simulink model "MPC_Experiments_2"  (R2020a)
settings: Solver=FixedStepAuto  StartTime=0.0  StopTime=tsim  FixedStep=baseRate  RelTol=1e-3  EnableMultiTasking=on
values from neighbouring files (symbols this model uses):
  Ad = dss.A    [theInitializer.m]
  ALGORITHM = 5    [Run_Initializer.m]    (also in main.m)
  baseRate = 0.05    [Run_Initializer.m]
  Bd = dss.B    [theInitializer.m]
  Cmat = zeros(6*N,9*N)    [theInitializer.m]
  con0 = [n*N, 2*N, N, N, N, N]    [Run_Initializer.m]    (also in main.m)
  drop_states_BLACK = rand([3,1])/10+init_states_BLACK    [Run_Initializer.m]
  drop_states_BLUE = rand([3,1])/10+init_states_BLUE    [Run_Initializer.m]
  drop_states_RED = rand([3,1])/10+init_states_RED    [Run_Initializer.m]
  F_thrusters_BLACK = 0.25.*ones(8,1)    [Run_Initializer.m]
  F_thrusters_BLUE = 0.25.*ones(8,1)    [Run_Initializer.m]
  F_thrusters_RED = 0.25.*ones(8,1)    [Run_Initializer.m]
  Fmat = reshape(repmat([umax,umax,taumax],N,1),3*N,1)    [theInitializer.m]
  gamma = 0.95    [theInitializer.m]
  H = blkdiag(pattern{:})    [theInitializer.m]
  home_states_BLACK = [ xLength/2; yLength/2; 0]    [Run_Initializer.m]
  home_states_BLUE = [ xLength/2-0.9; yLength/2+0.5; 0]    [Run_Initializer.m]
  home_states_RED = [ xLength/2+0.7; yLength/2; pi]    [Run_Initializer.m]
  init_states_BLACK = [ct;thetat0]    [Run_Initializer.m]
  init_states_BLUE = [pobj1;0]    [Run_Initializer.m]
  init_states_RED = xi(1:3)    [Run_Initializer.m]
  Kd_tb = 0.4    [Run_Initializer.m]
  Kd_tblue = 0.4    [Run_Initializer.m]
  Kd_tr = 0.4    [Run_Initializer.m]
  Kd_xb = 5    [Run_Initializer.m]
  Kd_xblue = 5    [Run_Initializer.m]
  Kd_xr = 5    [Run_Initializer.m]
  Kd_yb = 5    [Run_Initializer.m]
  Kd_yblue = 5    [Run_Initializer.m]
  Kd_yr = 5    [Run_Initializer.m]
  KOZ_actual = KOZ + rc*sqrt(2)    [theInitializer.m]
  Kp_tb = 0.1    [Run_Initializer.m]
  Kp_tblue = 0.1    [Run_Initializer.m]
  Kp_tr = 0.1    [Run_Initializer.m]
  Kp_xb = 2    [Run_Initializer.m]
  Kp_xblue = 2    [Run_Initializer.m]
  Kp_xr = 2    [Run_Initializer.m]
  Kp_yb = 2    [Run_Initializer.m]
  Kp_yblue = 2    [Run_Initializer.m]
  Kp_yr = 2    [Run_Initializer.m]
  N = 15    [Run_Initializer.m]    (also in main.m)
  noise_variance_BLACK = 0    [Run_Initializer.m]
  noise_variance_BLUE = 0    [Run_Initializer.m]
  noise_variance_RED = 0    [Run_Initializer.m]
  Phase0_End = Phase0_Duration    (= 5)    [Run_Initializer.m]
  Phase1_End = Phase0_Duration + Phase1_Duration    (= 10)    [Run_Initializer.m]
  Phase2_End = Phase0_Duration + Phase1_Duration +                                   Phase2_Duration    (= 36)    [Run_Initializer.m]
  Phase3_End = Phase0_Duration + Phase1_Duration +                                   Phase2_Duration + Phase3_Duration    (= 166)    [Run_Initializer.m]
  Phase3_SubPhase1_End = Phase2_End + Phase3_SubPhase1_Duration    (= 40)    [Run_Initializer.m]
  Phase3_SubPhase2_End = Phase2_End + Phase3_SubPhase1_Duration +                                   Phase3_SubPhase2_Duration    (= 42)    [Run_Initializer.m]
  Phase3_SubPhase3_End = Phase2_End + Phase3_SubPhase1_Duration +                                   Phase3_SubPhase2_Duration +                                  Phase3_SubPhase3_Duration    (= 44)    [Run_Initializer.m]
  Phase3_SubPhase4_End = Phase2_End + Phase3_SubPhase1_Duration +                                   Phase3_SubPhase2_Duration +                                  Phase3_SubPhase3_Duration +                                  Phase3_SubPhase4_Duration    [Run_Initializer.m]
  Phase4_End = Phase0_Duration + Phase1_Duration +                                   Phase2_Duration + Phase3_Duration +                                   Phase4_Duration    (= 186)    [Run_Initializer.m]
  Phase5_End = Phase0_Duration + Phase1_Duration +                                   Phase2_Duration + Phase3_Duration +                                   Phase4_Duration + Phase5_Duration    (= 191)    [Run_Initializer.m]
  pobj2 = [2.0; 0.5]    [Run_Initializer.m]    (also in main.m = pobj2hz(:,2); theNonlinearConstraints0.m = pobj2hz(:,i+2))
  Q = [10,0,0,0,0,0; 0,10,0,0,0,0; 0,0,10,0,0,0; 0,0,0,300,0,0; 0,0,0,0,300,0; 0,0,0,0,0,500]    [theInitializer.m]
  R = [10,0,0; 0,10,0; 0,0,10]    [theInitializer.m]
  rcone = 0.75    [theInitializer.m]
  rdock = rt+rc+wdock    (= 0.35)    [theInitializer.m]
  rt = 0.15    [theAnimatorExp.m]    (also in theInitializer.m)
  serverRate = 0.1    [Run_Initializer.m]
  Sj = [KOZ_actual^(-2),0; 0,KOZ_actual^(-2)]    [theInitializer.m]
  taumax = umax*rc    (= 0.0225)    [theInitializer.m]
  Td = 2    [Run_Initializer.m]    (also in main.m)
  thetah = 20.0 * d2r    (= 0.349065850399)    [theInitializer.m]
  thruster_dist2CG_BLACK = [83.42;-52.58;55.94;-60.05;54.08;-53.92;77.06;-55.94]    [Run_Initializer.m]
  thruster_dist2CG_BLUE = [83.42;-52.58;55.94;-60.05;54.08;-53.92;77.06;-55.94]    [Run_Initializer.m]
  thruster_dist2CG_RED = [49.92;-78.08;70.46;-63.54;81.08;-50.42;57.44;-75.96]    [Run_Initializer.m]
  tol = 0.0001    [Run_Initializer.m]    (also in main.m)
  Umat = zeros(3*N,9*N)    [theInitializer.m]
  umax = 0.15    [theInitializer.m]
  vobj2 = [0.0;0.0]    [Run_Initializer.m]    (also in main.m = [-0.02;-0.01])
undefined symbols (not defined in the file or in its folder): DiscIntNeverNeededParam, n, P, platformSelection, simMode, target_angular_velocity, WhoAmI
libraries: dspstat3 x18, raspberrypiBasiclib x10, dspsigops x9, embdlinuxlib x8, simulink x8, mspfiltlib x3, dsparch4 x3, dspswit3 x2, MainLibrary x2, sensehatlib x1
(part 5 of 10)

== system MPC_Experiments_2/Phase #3: Experiment/Change RED Behavior/Sub-Phase #1 ==
  note: ARM Control Law - RED
  note: PD Control Law - RED
  note: Additional Blocks
  note: Additional blocks are stored above. Note that to control attitude using the RW, simply replace RED_Tz with RED_Tz_RW.
  note: A simple PD control law is used here to command the platform to it's initial position, as defined in the initializer.
  note: This section is reserved for any control law for the robotic manipulator.
  Action Port : ActionPort  ActionPortLabel=if(u1 < u2)
  Constant{1,4..6} (4 alike) : Constant  Value=0
  Custom Discrete PD (Attitude) : Subsystem
  Custom Discrete PD (X-Position) : Subsystem
  Custom Discrete PD (Y-Position) : Subsystem
  Data Store Write : DataStoreWrite  DataStoreName=RED_Tz_Shoulder
  Data Store Write1 : DataStoreWrite  DataStoreName=RED_Tz_Elbow
  Data Store Write2 : DataStoreWrite  DataStoreName=RED_Tz_Wrist
  Data Store Write3 : DataStoreWrite  DataStoreName=Float_State
  Desired Attitude (RED) : Constant  Value=init_states_RED(3)  SampleTime=-1
  Desired X-Position (RED) : Constant  Value=init_states_RED(1)  SampleTime=-1
  Desired Y-Position (RED) : Constant  Value=init_states_RED(2)  SampleTime=-1
  Hough Control : Subsystem
  Puck State : Constant
  RED_Fx : DataStoreWrite  DataStoreName=RED_Fx
  RED_Fy : DataStoreWrite  DataStoreName=RED_Fy
  RED_Px : DataStoreRead  DataStoreName=RED_Px
  "RED_Py " : DataStoreRead  DataStoreName=RED_Py
  RED_Rz : DataStoreRead  DataStoreName=RED_Rz
  RED_Tz : DataStoreWrite  DataStoreName=RED_Tz
  RED_Tz_RW : DataStoreWrite  DataStoreName=RED_Tz_RW
  Subtract : Sum  Inputs=+-
  Subtract1 : Sum  Inputs=+-
  wires:
  Constant1/1 -> RED_Tz_RW/1
  Constant6/1 -> Data Store Write2/1
  Constant4/1 -> Data Store Write/1
  Constant5/1 -> Data Store Write1/1
  Desired Y-Position (RED)/1 -> Subtract1/1
  Custom Discrete PD (X-Position)/1(Fx) -> RED_Fx/1
  RED_Px/1 -> Subtract/2
  Desired Attitude (RED)/1 -> Hough Control/1(Ref)
  RED_Rz/1 -> Hough Control/2(Act)
  Custom Discrete PD (Y-Position)/1(Fy) -> RED_Fy/1
  Subtract1/1 -> Custom Discrete PD (Y-Position)/1(ey)
  "RED_Py "/1 -> Subtract1/2
  Subtract/1 -> Custom Discrete PD (X-Position)/1(ex)
  Hough Control/1(Err) -> Custom Discrete PD (Attitude)/1(ez)
  Custom Discrete PD (Attitude)/1(Tz) -> RED_Tz/1
  Desired X-Position (RED)/1 -> Subtract/1
  Puck State/1 -> Data Store Write3/1

== system MPC_Experiments_2/Phase #3: Experiment/Change RED Behavior/Sub-Phase #2  ==
  note: ARM Control Law - RED
  note: PD Control Law - RED
  note: Additional Blocks
  note: Additional blocks are stored above. Note that to control attitude using the RW, simply replace RED_Tz with RED_Tz_RW.
  note: This section is reserved for any control law for the robotic manipulator.
  Action Port : ActionPort  ActionPortLabel=elseif(u1 < u3)
  Constant{,1,4..6} (5 alike) : Constant  Value=0
  Data Store Write : DataStoreWrite  DataStoreName=RED_Tz_Shoulder
  Data Store Write1 : DataStoreWrite  DataStoreName=RED_Tz_Elbow
  Data Store Write2 : DataStoreWrite  DataStoreName=RED_Tz_Wrist
  Data Store Write3 : DataStoreWrite  DataStoreName=Float_State
  Puck State : Constant  Value=0
  RED_Fx : DataStoreWrite  DataStoreName=RED_Fx
  RED_Fy : DataStoreWrite  DataStoreName=RED_Fy
  RED_Tz : DataStoreWrite  DataStoreName=RED_Tz
  RED_Tz_RW : DataStoreWrite  DataStoreName=RED_Tz_RW
  wires:
  Constant1/1 -> RED_Tz_RW/1
  Constant6/1 -> Data Store Write2/1
  Constant4/1 -> Data Store Write/1
  Constant5/1 -> Data Store Write1/1
  Constant/1 -> RED_Tz/1, RED_Fx/1, RED_Fy/1
  Puck State/1 -> Data Store Write3/1

== system MPC_Experiments_2/Phase #3: Experiment/Change RED Behavior/Sub-Phase #3  ==
  note: ARM Control Law - RED
  note: PD Control Law - RED
  note: Additional Blocks
  note: Additional blocks are stored above. Note that to control attitude using the RW, simply replace RED_Tz with RED_Tz_RW.
  note: This section is reserved for any control law for the robotic manipulator.
  Action Port : ActionPort  ActionPortLabel=elseif( u1 < u4)
  Constant{,1,4..6} (5 alike) : Constant  Value=0
  Data Store Write : DataStoreWrite  DataStoreName=RED_Tz_Shoulder
  Data Store Write1 : DataStoreWrite  DataStoreName=RED_Tz_Elbow
  Data Store Write2 : DataStoreWrite  DataStoreName=RED_Tz_Wrist
  Data Store Write3 : DataStoreWrite  DataStoreName=Float_State
  Puck State : Constant
  RED_Fx : DataStoreWrite  DataStoreName=RED_Fx
  RED_Fy : DataStoreWrite  DataStoreName=RED_Fy
  RED_Tz : DataStoreWrite  DataStoreName=RED_Tz
  RED_Tz_RW : DataStoreWrite  DataStoreName=RED_Tz_RW
  wires:
  Constant1/1 -> RED_Tz_RW/1
  Constant6/1 -> Data Store Write2/1
  Constant4/1 -> Data Store Write/1
  Constant5/1 -> Data Store Write1/1
  Constant/1 -> RED_Tz/1, RED_Fx/1, RED_Fy/1
  Puck State/1 -> Data Store Write3/1

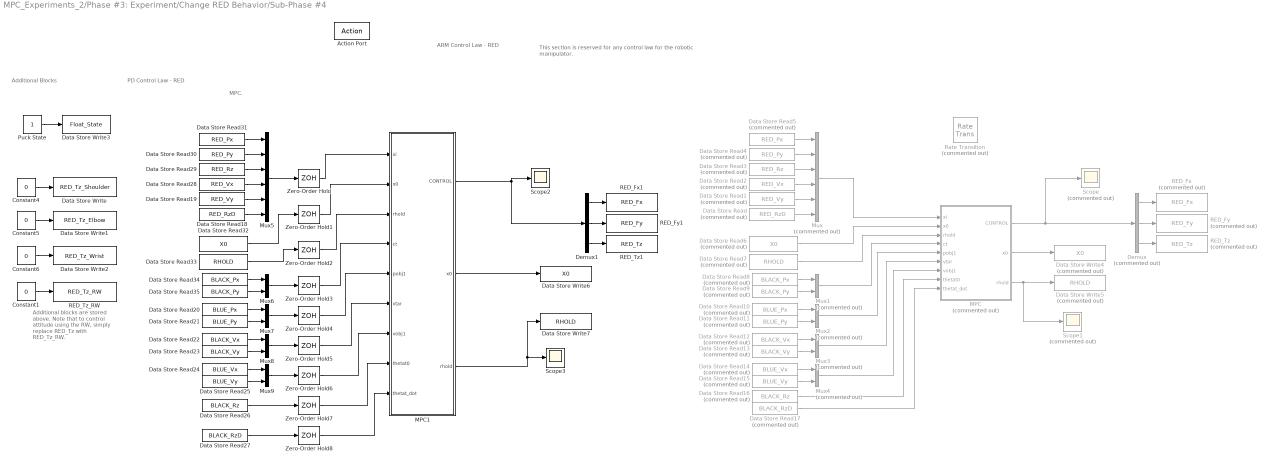
== system MPC_Experiments_2/Phase #3: Experiment/Change RED Behavior/Sub-Phase #4 ==
  note: ARM Control Law - RED
  note: PD Control Law - RED
  note: Additional Blocks
  note: Additional blocks are stored above. Note that to control attitude using the RW, simply replace RED_Tz with RED_Tz_RW.
  note: MPC.
  note: This section is reserved for any control law for the robotic manipulator.
  Action Port : ActionPort  ActionPortLabel=elseif( u1 < u5)
  Constant{1,4..6} (4 alike) : Constant  Value=0
  Data Store Read : DataStoreRead  Commented=on  DataStoreName=RED_RzD
  Data Store Read1 : DataStoreRead  Commented=on  DataStoreName=RED_Vy
  Data Store Read10 : DataStoreRead  Commented=on  DataStoreName=BLUE_Px
  Data Store Read11 : DataStoreRead  Commented=on  DataStoreName=BLUE_Py
  Data Store Read12 : DataStoreRead  Commented=on  DataStoreName=BLACK_Vx
  Data Store Read13 : DataStoreRead  Commented=on  DataStoreName=BLACK_Vy
  Data Store Read14 : DataStoreRead  Commented=on  DataStoreName=BLUE_Vx
  Data Store Read15 : DataStoreRead  Commented=on  DataStoreName=BLUE_Vy
  Data Store Read16 : DataStoreRead  Commented=on  DataStoreName=BLACK_Rz
  Data Store Read17 : DataStoreRead  Commented=on  DataStoreName=BLACK_RzD
  Data Store Read18 : DataStoreRead  DataStoreName=RED_RzD
  Data Store Read19 : DataStoreRead  DataStoreName=RED_Vy
  Data Store Read2 : DataStoreRead  Commented=on  DataStoreName=RED_Vx
  Data Store Read20 : DataStoreRead  DataStoreName=BLUE_Px
  Data Store Read21 : DataStoreRead  DataStoreName=BLUE_Py
  Data Store Read22 : DataStoreRead  DataStoreName=BLACK_Vx
  Data Store Read23 : DataStoreRead  DataStoreName=BLACK_Vy
  Data Store Read24 : DataStoreRead  DataStoreName=BLUE_Vx
  Data Store Read25 : DataStoreRead  DataStoreName=BLUE_Vy
  Data Store Read26 : DataStoreRead  DataStoreName=BLACK_Rz
  Data Store Read27 : DataStoreRead  DataStoreName=BLACK_RzD
  Data Store Read28 : DataStoreRead  DataStoreName=RED_Vx
  Data Store Read29 : DataStoreRead  DataStoreName=RED_Rz
  Data Store Read3 : DataStoreRead  Commented=on  DataStoreName=RED_Rz
  Data Store Read30 : DataStoreRead  DataStoreName=RED_Py
  Data Store Read31 : DataStoreRead  DataStoreName=RED_Px
  Data Store Read32 : DataStoreRead  DataStoreName=X0
  Data Store Read33 : DataStoreRead  DataStoreName=RHOLD
  Data Store Read34 : DataStoreRead  DataStoreName=BLACK_Px
  Data Store Read35 : DataStoreRead  DataStoreName=BLACK_Py
  Data Store Read4 : DataStoreRead  Commented=on  DataStoreName=RED_Py
  Data Store Read5 : DataStoreRead  Commented=on  DataStoreName=RED_Px
  Data Store Read6 : DataStoreRead  Commented=on  DataStoreName=X0
  Data Store Read7 : DataStoreRead  Commented=on  DataStoreName=RHOLD
  Data Store Read8 : DataStoreRead  Commented=on  DataStoreName=BLACK_Px
  Data Store Read9 : DataStoreRead  Commented=on  DataStoreName=BLACK_Py
  Data Store Write : DataStoreWrite  DataStoreName=RED_Tz_Shoulder
  Data Store Write1 : DataStoreWrite  DataStoreName=RED_Tz_Elbow
  Data Store Write2 : DataStoreWrite  DataStoreName=RED_Tz_Wrist
  Data Store Write3 : DataStoreWrite  DataStoreName=Float_State
  Data Store Write4 : DataStoreWrite  Commented=on  DataStoreName=X0
  Data Store Write5 : DataStoreWrite  Commented=on  DataStoreName=RHOLD
  Data Store Write6 : DataStoreWrite  DataStoreName=X0
  Data Store Write7 : DataStoreWrite  DataStoreName=RHOLD
  Demux : Demux  Commented=on  Outputs=3
  Demux1 : Demux  Outputs=3
  MPC : MATLAB Function  Commented=on  TreatAsAtomicUnit=on  SystemSampleTime=Td
  MPC1 : MATLAB Function  TreatAsAtomicUnit=on
  Mux : Mux  Commented=on  Inputs=6
  Mux{1..4} (4 alike) : Mux  Commented=on  Inputs=2
  Mux5 : Mux  Inputs=6
  Mux{6..9} (4 alike) : Mux  Inputs=2
  Puck State : Constant
  RED_Fx : DataStoreWrite  Commented=on  DataStoreName=RED_Fx
  RED_Fx1 : DataStoreWrite  DataStoreName=RED_Fx
  RED_Fy : DataStoreWrite  Commented=on  DataStoreName=RED_Fy
  RED_Fy1 : DataStoreWrite  DataStoreName=RED_Fy
  RED_Tz : DataStoreWrite  Commented=on  DataStoreName=RED_Tz
  RED_Tz1 : DataStoreWrite  DataStoreName=RED_Tz
  RED_Tz_RW : DataStoreWrite  DataStoreName=RED_Tz_RW
  Rate Transition : RateTransition  Commented=on
  Scope : Scope  Commented=on
  Scope1 : Scope  Commented=on
  Scope2 : Scope
  Scope3 : Scope
  Zero-Order Hold{,1..8} (9 alike) : ZeroOrderHold  SampleTime=Td
  wires:
  Constant1/1 -> RED_Tz_RW/1
  Constant6/1 -> Data Store Write2/1
  Constant4/1 -> Data Store Write/1
  Constant5/1 -> Data Store Write1/1
  Puck State/1 -> Data Store Write3/1
  Data Store Read1/1 -> Mux/5
  Data Store Read5/1 -> Mux/1
  Data Store Read4/1 -> Mux/2
  Data Store Read7/1 -> MPC/3("rhold ")
  Demux/3 -> RED_Tz/1
  MPC/2(x0) -> Data Store Write4/1
  MPC/3(rhold) -> Data Store Write5/1, Scope1/1
  Demux/2 -> RED_Fy/1
  Data Store Read6/1 -> MPC/2("x0 ")
  Mux/1 -> MPC/1(xi)
  Data Store Read/1 -> Mux/6
  Demux/1 -> RED_Fx/1
  Data Store Read2/1 -> Mux/4
  MPC/1(CONTROL) -> Scope/1, Demux/1
  Data Store Read3/1 -> Mux/3
  Data Store Read8/1 -> Mux1/1
  Data Store Read9/1 -> Mux1/2
  Data Store Read10/1 -> Mux2/1
  Data Store Read11/1 -> Mux2/2
  Mux1/1 -> MPC/4(ct)
  Mux2/1 -> MPC/5(pobj1)
  Data Store Read12/1 -> Mux3/1
  Data Store Read13/1 -> Mux3/2
  Mux3/1 -> MPC/6(vtar)
  Data Store Read14/1 -> Mux4/1
  Data Store Read15/1 -> Mux4/2
  Mux4/1 -> MPC/7(vobj1)
  Data Store Read16/1 -> MPC/8(thetat0)
  Data Store Read17/1 -> MPC/9(thetat_dot)
  MPC1/3(rhold) -> Data Store Write7/1, Scope3/1
  Mux8/1 -> Zero-Order Hold5/1
  Zero-Order Hold5/1 -> MPC1/6(vtar)
  Zero-Order Hold8/1 -> MPC1/9(thetat_dot)
  MPC1/2(x0) -> Data Store Write6/1
  Zero-Order Hold3/1 -> MPC1/4(ct)
  Zero-Order Hold6/1 -> MPC1/7(vobj1)
  Data Store Read32/1 -> Zero-Order Hold1/1
  Zero-Order Hold/1 -> MPC1/1(xi)
  Zero-Order Hold4/1 -> MPC1/5(pobj1)
  Demux1/1 -> RED_Fx1/1
  Data Store Read29/1 -> Mux5/3
  Data Store Read22/1 -> Mux8/1
  Data Store Read35/1 -> Mux6/2
  Zero-Order Hold2/1 -> MPC1/3("rhold ")
  Data Store Read20/1 -> Mux7/1
  Zero-Order Hold1/1 -> MPC1/2("x0 ")
  Zero-Order Hold7/1 -> MPC1/8(thetat0)
  Mux7/1 -> Zero-Order Hold4/1
  Data Store Read21/1 -> Mux7/2
  Data Store Read30/1 -> Mux5/2
  Demux1/2 -> RED_Fy1/1
  Data Store Read27/1 -> Zero-Order Hold8/1
  Mux9/1 -> Zero-Order Hold6/1
  Mux6/1 -> Zero-Order Hold3/1
  Data Store Read24/1 -> Mux9/1
  Mux5/1 -> Zero-Order Hold/1
  Data Store Read28/1 -> Mux5/4
  Data Store Read34/1 -> Mux6/1
  Demux1/3 -> RED_Tz1/1
  Data Store Read25/1 -> Mux9/2
  Data Store Read18/1 -> Mux5/6
  Data Store Read26/1 -> Zero-Order Hold7/1
  Data Store Read23/1 -> Mux8/2
  Data Store Read33/1 -> Zero-Order Hold2/1
  Data Store Read19/1 -> Mux5/5
  Data Store Read31/1 -> Mux5/1
  MPC1/1(CONTROL) -> Scope2/1, Demux1/1

== system MPC_Experiments_2/Phase #3: Experiment/Change RED Behavior/Subsystem ==
  Universal_Time : DataStoreRead  DataStoreName=Univ_Time
  Time : Outport  VectorParamsAs1DForOutWhenUnconnected=off
  wires:
  Universal_Time/1 -> Time/1

== system MPC_Experiments_2/Phase #4: Return Home/Change BLACK Behavior/Custom Discrete PD (Attitude) ==
  ez : Inport
  Sum3 : Sum
  kd_tb : Gain  Gain=Kd_tb
  kp_tb : Gain  Gain=Kp_tb
  "x_dot -> x1" : Subsystem
  Tz : Outport  VectorParamsAs1DForOutWhenUnconnected=off
  wires:
  kd_tb/1 -> Sum3/1
  Sum3/1 -> Tz/1
  kp_tb/1 -> Sum3/2
  "x_dot -> x1"/1(dy(t)/dt) -> kd_tb/1
  ez/1 -> "x_dot -> x1"/1(y(t)), kp_tb/1

== system MPC_Experiments_2/Phase #4: Return Home/Change BLACK Behavior/Custom Discrete PD (X-Position) ==
  ex : Inport
  Sum3 : Sum
  kd_xb : Gain  Gain=Kd_xb
  kp_xb : Gain  Gain=Kp_xb
  "x_dot -> x1" : Subsystem
  Fx : Outport  VectorParamsAs1DForOutWhenUnconnected=off
  wires:
  kd_xb/1 -> Sum3/1
  ex/1 -> "x_dot -> x1"/1(y(t)), kp_xb/1
  kp_xb/1 -> Sum3/2
  "x_dot -> x1"/1(dy(t)/dt) -> kd_xb/1
  Sum3/1 -> Fx/1

== system MPC_Experiments_2/Phase #4: Return Home/Change BLACK Behavior/Custom Discrete PD (Y-Position) ==
  ey : Inport
  Sum3 : Sum
  kd_yb : Gain  Gain=Kd_yb
  kp_yb : Gain  Gain=Kp_yb
  "x_dot -> x1" : Subsystem
  Fy : Outport  VectorParamsAs1DForOutWhenUnconnected=off
  wires:
  kd_yb/1 -> Sum3/1
  Sum3/1 -> Fy/1
  kp_yb/1 -> Sum3/2
  "x_dot -> x1"/1(dy(t)/dt) -> kd_yb/1
  ey/1 -> "x_dot -> x1"/1(y(t)), kp_yb/1

== system MPC_Experiments_2/Phase #4: Return Home/Change BLACK Behavior/Hough Control ==
  Ref : Inport
  Act : Inport  Port=2
  MATLAB Function2 : MATLAB Function  TreatAsAtomicUnit=on
  MATLAB Function3 : MATLAB Function  TreatAsAtomicUnit=on
  MATLAB Function4 : MATLAB Function  TreatAsAtomicUnit=on
  Subtract2 : Sum  Inputs=+-
  Err : Outport  VectorParamsAs1DForOutWhenUnconnected=off
  wires:
  MATLAB Function4/1(e_out) -> Err/1
  MATLAB Function2/1(Oy) -> MATLAB Function4/1(Oy)
  Subtract2/1 -> MATLAB Function4/2(e_in)
  MATLAB Function2/2(Ox) -> Subtract2/1
  Act/1 -> MATLAB Function3/1(z)
  Ref/1 -> MATLAB Function2/1(z)
  MATLAB Function3/1(Ox) -> Subtract2/2

== system MPC_Experiments_2/Phase #4: Return Home/Change BLUE Behavior/Custom Discrete PD (Attitude) ==
  ez : Inport
  Sum3 : Sum
  kd_tb : Gain  Gain=Kd_tblue
  kp_tb : Gain  Gain=Kp_tblue
  "x_dot -> x1" : Subsystem
  Tz : Outport  VectorParamsAs1DForOutWhenUnconnected=off
  wires:
  kd_tb/1 -> Sum3/1
  Sum3/1 -> Tz/1
  kp_tb/1 -> Sum3/2
  "x_dot -> x1"/1(dy(t)/dt) -> kd_tb/1
  ez/1 -> "x_dot -> x1"/1(y(t)), kp_tb/1

== system MPC_Experiments_2/Phase #4: Return Home/Change BLUE Behavior/Custom Discrete PD (X-Position) ==
  ex : Inport
  Sum3 : Sum
  kd_xb : Gain  Gain=Kd_xblue
  kp_xb : Gain  Gain=Kp_xblue
  "x_dot -> x1" : Subsystem
  Fx : Outport  VectorParamsAs1DForOutWhenUnconnected=off
  wires:
  kd_xb/1 -> Sum3/1
  ex/1 -> "x_dot -> x1"/1(y(t)), kp_xb/1
  kp_xb/1 -> Sum3/2
  "x_dot -> x1"/1(dy(t)/dt) -> kd_xb/1
  Sum3/1 -> Fx/1

== system MPC_Experiments_2/Phase #4: Return Home/Change BLUE Behavior/Custom Discrete PD (Y-Position) ==
  ey : Inport
  Sum3 : Sum
  kd_yb : Gain  Gain=Kd_yblue
  kp_yb : Gain  Gain=Kp_yblue
  "x_dot -> x1" : Subsystem
  Fy : Outport  VectorParamsAs1DForOutWhenUnconnected=off
  wires:
  kd_yb/1 -> Sum3/1
  Sum3/1 -> Fy/1
  kp_yb/1 -> Sum3/2
  "x_dot -> x1"/1(dy(t)/dt) -> kd_yb/1
  ey/1 -> "x_dot -> x1"/1(y(t)), kp_yb/1

== system MPC_Experiments_2/Phase #4: Return Home/Change BLUE Behavior/Hough Control ==
  Ref : Inport
  Act : Inport  Port=2
  MATLAB Function2 : MATLAB Function  TreatAsAtomicUnit=on
  MATLAB Function3 : MATLAB Function  TreatAsAtomicUnit=on
  MATLAB Function4 : MATLAB Function  TreatAsAtomicUnit=on
  Subtract2 : Sum  Inputs=+-
  Err : Outport  VectorParamsAs1DForOutWhenUnconnected=off
  wires:
  MATLAB Function4/1(e_out) -> Err/1
  MATLAB Function2/1(Oy) -> MATLAB Function4/1(Oy)
  Subtract2/1 -> MATLAB Function4/2(e_in)
  MATLAB Function2/2(Ox) -> Subtract2/1
  Act/1 -> MATLAB Function3/1(z)
  Ref/1 -> MATLAB Function2/1(z)
  MATLAB Function3/1(Ox) -> Subtract2/2

== system MPC_Experiments_2/Phase #4: Return Home/Change RED Behavior/Custom Discrete PD (Attitude) ==
  ez : Inport
  Sum3 : Sum
  kd_tr : Gain  Gain=Kd_tr
  kp_tr : Gain  Gain=Kp_tr
  "x_dot -> x1" : Subsystem
  Tz : Outport  VectorParamsAs1DForOutWhenUnconnected=off
  wires:
  kd_tr/1 -> Sum3/1
  Sum3/1 -> Tz/1
  kp_tr/1 -> Sum3/2
  "x_dot -> x1"/1(dy(t)/dt) -> kd_tr/1
  ez/1 -> "x_dot -> x1"/1(y(t)), kp_tr/1

== system MPC_Experiments_2/Phase #4: Return Home/Change RED Behavior/Custom Discrete PD (X-Position) ==
  ex : Inport
  Sum3 : Sum
  kd_xr : Gain  Gain=Kd_xr
  kp_xr : Gain  Gain=Kp_xr
  "x_dot -> x1" : Subsystem
  Fx : Outport  VectorParamsAs1DForOutWhenUnconnected=off
  wires:
  kd_xr/1 -> Sum3/1
  ex/1 -> "x_dot -> x1"/1(y(t)), kp_xr/1
  kp_xr/1 -> Sum3/2
  "x_dot -> x1"/1(dy(t)/dt) -> kd_xr/1
  Sum3/1 -> Fx/1

== system MPC_Experiments_2/Phase #4: Return Home/Change RED Behavior/Custom Discrete PD (Y-Position) ==
  ey : Inport
  Sum3 : Sum
  kd_yr : Gain  Gain=Kd_yr
  kp_yr : Gain  Gain=Kp_yr
  "x_dot -> x1" : Subsystem
  Fy : Outport  VectorParamsAs1DForOutWhenUnconnected=off
  wires:
  kd_yr/1 -> Sum3/1
  Sum3/1 -> Fy/1
  kp_yr/1 -> Sum3/2
  "x_dot -> x1"/1(dy(t)/dt) -> kd_yr/1
  ey/1 -> "x_dot -> x1"/1(y(t)), kp_yr/1

== system MPC_Experiments_2/Phase #4: Return Home/Change RED Behavior/Hough Control ==
  Ref : Inport
  Act : Inport  Port=2
  MATLAB Function2 : MATLAB Function  TreatAsAtomicUnit=on
  MATLAB Function3 : MATLAB Function  TreatAsAtomicUnit=on
  MATLAB Function4 : MATLAB Function  TreatAsAtomicUnit=on
  Subtract2 : Sum  Inputs=+-
  Err : Outport  VectorParamsAs1DForOutWhenUnconnected=off
  wires:
  MATLAB Function4/1(e_out) -> Err/1
  MATLAB Function2/1(Oy) -> MATLAB Function4/1(Oy)
  Subtract2/1 -> MATLAB Function4/2(e_in)
  MATLAB Function2/2(Ox) -> Subtract2/1
  Act/1 -> MATLAB Function3/1(z)
  Ref/1 -> MATLAB Function2/1(z)
  MATLAB Function3/1(Ox) -> Subtract2/2

== system MPC_Experiments_2/Phase #5: Hold Home/Change BLACK Behavior/Custom Discrete PD (Attitude) ==
  ez : Inport
  Sum3 : Sum
  kd_tb : Gain  Gain=Kd_tb
  kp_tb : Gain  Gain=Kp_tb
  "x_dot -> x1" : Subsystem
  Tz : Outport  VectorParamsAs1DForOutWhenUnconnected=off
  wires:
  kd_tb/1 -> Sum3/1
  Sum3/1 -> Tz/1
  kp_tb/1 -> Sum3/2
  "x_dot -> x1"/1(dy(t)/dt) -> kd_tb/1
  ez/1 -> "x_dot -> x1"/1(y(t)), kp_tb/1

== system MPC_Experiments_2/Phase #5: Hold Home/Change BLACK Behavior/Custom Discrete PD (X-Position) ==
  ex : Inport
  Sum3 : Sum
  kd_xb : Gain  Gain=Kd_xb
  kp_xb : Gain  Gain=Kp_xb
  "x_dot -> x1" : Subsystem
  Fx : Outport  VectorParamsAs1DForOutWhenUnconnected=off
  wires:
  kd_xb/1 -> Sum3/1
  ex/1 -> "x_dot -> x1"/1(y(t)), kp_xb/1
  kp_xb/1 -> Sum3/2
  "x_dot -> x1"/1(dy(t)/dt) -> kd_xb/1
  Sum3/1 -> Fx/1

== system MPC_Experiments_2/Phase #5: Hold Home/Change BLACK Behavior/Custom Discrete PD (Y-Position) ==
  ey : Inport
  Sum3 : Sum
  kd_yb : Gain  Gain=Kd_yb
  kp_yb : Gain  Gain=Kp_yb
  "x_dot -> x1" : Subsystem
  Fy : Outport  VectorParamsAs1DForOutWhenUnconnected=off
  wires:
  kd_yb/1 -> Sum3/1
  Sum3/1 -> Fy/1
  kp_yb/1 -> Sum3/2
  "x_dot -> x1"/1(dy(t)/dt) -> kd_yb/1
  ey/1 -> "x_dot -> x1"/1(y(t)), kp_yb/1

== system MPC_Experiments_2/Phase #5: Hold Home/Change BLACK Behavior/Hough Control ==
  Ref : Inport
  Act : Inport  Port=2
  MATLAB Function2 : MATLAB Function  TreatAsAtomicUnit=on
  MATLAB Function3 : MATLAB Function  TreatAsAtomicUnit=on
  MATLAB Function4 : MATLAB Function  TreatAsAtomicUnit=on
  Subtract2 : Sum  Inputs=+-
  Err : Outport  VectorParamsAs1DForOutWhenUnconnected=off
  wires:
  MATLAB Function4/1(e_out) -> Err/1
  MATLAB Function2/1(Oy) -> MATLAB Function4/1(Oy)
  Subtract2/1 -> MATLAB Function4/2(e_in)
  MATLAB Function2/2(Ox) -> Subtract2/1
  Act/1 -> MATLAB Function3/1(z)
  Ref/1 -> MATLAB Function2/1(z)
  MATLAB Function3/1(Ox) -> Subtract2/2

== system MPC_Experiments_2/Phase #5: Hold Home/Change BLUE Behavior/Custom Discrete PD (Attitude) ==
  ez : Inport
  Sum3 : Sum
  kd_tb : Gain  Gain=Kd_tblue
  kp_tb : Gain  Gain=Kp_tblue
  "x_dot -> x1" : Subsystem
  Tz : Outport  VectorParamsAs1DForOutWhenUnconnected=off
  wires:
  kd_tb/1 -> Sum3/1
  Sum3/1 -> Tz/1
  kp_tb/1 -> Sum3/2
  "x_dot -> x1"/1(dy(t)/dt) -> kd_tb/1
  ez/1 -> "x_dot -> x1"/1(y(t)), kp_tb/1

== system MPC_Experiments_2/Phase #5: Hold Home/Change BLUE Behavior/Custom Discrete PD (X-Position) ==
  ex : Inport
  Sum3 : Sum
  kd_xb : Gain  Gain=Kd_xblue
  kp_xb : Gain  Gain=Kp_xblue
  "x_dot -> x1" : Subsystem
  Fx : Outport  VectorParamsAs1DForOutWhenUnconnected=off
  wires:
  kd_xb/1 -> Sum3/1
  ex/1 -> "x_dot -> x1"/1(y(t)), kp_xb/1
  kp_xb/1 -> Sum3/2
  "x_dot -> x1"/1(dy(t)/dt) -> kd_xb/1
  Sum3/1 -> Fx/1

== system MPC_Experiments_2/Phase #5: Hold Home/Change BLUE Behavior/Custom Discrete PD (Y-Position) ==
  ey : Inport
  Sum3 : Sum
  kd_yb : Gain  Gain=Kd_yblue
  kp_yb : Gain  Gain=Kp_yblue
  "x_dot -> x1" : Subsystem
  Fy : Outport  VectorParamsAs1DForOutWhenUnconnected=off
  wires:
  kd_yb/1 -> Sum3/1
  Sum3/1 -> Fy/1
  kp_yb/1 -> Sum3/2
  "x_dot -> x1"/1(dy(t)/dt) -> kd_yb/1
  ey/1 -> "x_dot -> x1"/1(y(t)), kp_yb/1

== system MPC_Experiments_2/Phase #5: Hold Home/Change BLUE Behavior/Hough Control ==
  Ref : Inport
  Act : Inport  Port=2
  MATLAB Function2 : MATLAB Function  TreatAsAtomicUnit=on
  MATLAB Function3 : MATLAB Function  TreatAsAtomicUnit=on
  MATLAB Function4 : MATLAB Function  TreatAsAtomicUnit=on
  Subtract2 : Sum  Inputs=+-
  Err : Outport  VectorParamsAs1DForOutWhenUnconnected=off
  wires:
  MATLAB Function4/1(e_out) -> Err/1
  MATLAB Function2/1(Oy) -> MATLAB Function4/1(Oy)
  Subtract2/1 -> MATLAB Function4/2(e_in)
  MATLAB Function2/2(Ox) -> Subtract2/1
  Act/1 -> MATLAB Function3/1(z)
  Ref/1 -> MATLAB Function2/1(z)
  MATLAB Function3/1(Ox) -> Subtract2/2

== system MPC_Experiments_2/Phase #5: Hold Home/Change RED Behavior/Custom Discrete PD (Attitude) ==
  ez : Inport
  Sum3 : Sum
  kd_tr : Gain  Gain=Kd_tr
  kp_tr : Gain  Gain=Kp_tr
  "x_dot -> x1" : Subsystem
  Tz : Outport  VectorParamsAs1DForOutWhenUnconnected=off
  wires:
  kd_tr/1 -> Sum3/1
  Sum3/1 -> Tz/1
  kp_tr/1 -> Sum3/2
  "x_dot -> x1"/1(dy(t)/dt) -> kd_tr/1
  ez/1 -> "x_dot -> x1"/1(y(t)), kp_tr/1

== system MPC_Experiments_2/Phase #5: Hold Home/Change RED Behavior/Custom Discrete PD (X-Position) ==
  ex : Inport
  Sum3 : Sum
  kd_xr : Gain  Gain=Kd_xr
  kp_xr : Gain  Gain=Kp_xr
  "x_dot -> x1" : Subsystem
  Fx : Outport  VectorParamsAs1DForOutWhenUnconnected=off
  wires:
  kd_xr/1 -> Sum3/1
  ex/1 -> "x_dot -> x1"/1(y(t)), kp_xr/1
  kp_xr/1 -> Sum3/2
  "x_dot -> x1"/1(dy(t)/dt) -> kd_xr/1
  Sum3/1 -> Fx/1

== system MPC_Experiments_2/Phase #5: Hold Home/Change RED Behavior/Custom Discrete PD (Y-Position) ==
  ey : Inport
  Sum3 : Sum
  kd_yr : Gain  Gain=Kd_yr
  kp_yr : Gain  Gain=Kp_yr
  "x_dot -> x1" : Subsystem
  Fy : Outport  VectorParamsAs1DForOutWhenUnconnected=off
  wires:
  kd_yr/1 -> Sum3/1
  Sum3/1 -> Fy/1
  kp_yr/1 -> Sum3/2
  "x_dot -> x1"/1(dy(t)/dt) -> kd_yr/1
  ey/1 -> "x_dot -> x1"/1(y(t)), kp_yr/1

== system MPC_Experiments_2/Phase #5: Hold Home/Change RED Behavior/Hough Control ==
  Ref : Inport
  Act : Inport  Port=2
  MATLAB Function2 : MATLAB Function  TreatAsAtomicUnit=on
  MATLAB Function3 : MATLAB Function  TreatAsAtomicUnit=on
  MATLAB Function4 : MATLAB Function  TreatAsAtomicUnit=on
  Subtract2 : Sum  Inputs=+-
  Err : Outport  VectorParamsAs1DForOutWhenUnconnected=off
  wires:
  MATLAB Function4/1(e_out) -> Err/1
  MATLAB Function2/1(Oy) -> MATLAB Function4/1(Oy)
  Subtract2/1 -> MATLAB Function4/2(e_in)
  MATLAB Function2/2(Ox) -> Subtract2/1
  Act/1 -> MATLAB Function3/1(z)
  Ref/1 -> MATLAB Function2/1(z)
  MATLAB Function3/1(Ox) -> Subtract2/2

== system MPC_Experiments_2/Simulate Plant Dynamics/x_dot -> x1/Hold this value ==
  In1 : Inport
  Action Port : ActionPort  ActionPortLabel=if(u1 ~= 0)
  Out1 : Outport  VectorParamsAs1DForOutWhenUnconnected=off
  wires:
  In1/1 -> Out1/1

== system MPC_Experiments_2/Simulate Plant Dynamics/x_dot -> x10/Hold this value ==
  In1 : Inport
  Action Port : ActionPort  ActionPortLabel=if(u1 ~= 0)
  Out1 : Outport  VectorParamsAs1DForOutWhenUnconnected=off
  wires:
  In1/1 -> Out1/1

== system MPC_Experiments_2/Simulate Plant Dynamics/x_dot -> x11/Hold this value ==
  In1 : Inport
  Action Port : ActionPort  ActionPortLabel=if(u1 ~= 0)
  Out1 : Outport  VectorParamsAs1DForOutWhenUnconnected=off
  wires:
  In1/1 -> Out1/1

== system MPC_Experiments_2/Simulate Plant Dynamics/x_dot -> x13/Hold this value ==
  In1 : Inport
  Action Port : ActionPort  ActionPortLabel=if(u1 ~= 0)
  Out1 : Outport  VectorParamsAs1DForOutWhenUnconnected=off
  wires:
  In1/1 -> Out1/1

== system MPC_Experiments_2/Simulate Plant Dynamics/x_dot -> x14/Hold this value ==
  In1 : Inport
  Action Port : ActionPort  ActionPortLabel=if(u1 ~= 0)
  Out1 : Outport  VectorParamsAs1DForOutWhenUnconnected=off
  wires:
  In1/1 -> Out1/1

== system MPC_Experiments_2/Simulate Plant Dynamics/x_dot -> x16/Hold this value ==
  In1 : Inport
  Action Port : ActionPort  ActionPortLabel=if(u1 ~= 0)
  Out1 : Outport  VectorParamsAs1DForOutWhenUnconnected=off
  wires:
  In1/1 -> Out1/1

== system MPC_Experiments_2/Simulate Plant Dynamics/x_dot -> x17/Hold this value ==
  In1 : Inport
  Action Port : ActionPort  ActionPortLabel=if(u1 ~= 0)
  Out1 : Outport  VectorParamsAs1DForOutWhenUnconnected=off
  wires:
  In1/1 -> Out1/1

== system MPC_Experiments_2/Simulate Plant Dynamics/x_dot -> x2/Hold this value ==
  In1 : Inport
  Action Port : ActionPort  ActionPortLabel=if(u1 ~= 0)
  Out1 : Outport  VectorParamsAs1DForOutWhenUnconnected=off
  wires:
  In1/1 -> Out1/1

== system MPC_Experiments_2/Simulate Plant Dynamics/x_dot -> x3/Hold this value ==
  In1 : Inport
  Action Port : ActionPort  ActionPortLabel=if(u1 ~= 0)
  Out1 : Outport  VectorParamsAs1DForOutWhenUnconnected=off
  wires:
  In1/1 -> Out1/1

== system MPC_Experiments_2/Simulate Plant Dynamics/x_dot -> x4/Hold this value ==
  In1 : Inport
  Action Port : ActionPort  ActionPortLabel=if(u1 ~= 0)
  Out1 : Outport  VectorParamsAs1DForOutWhenUnconnected=off
  wires:
  In1/1 -> Out1/1

== system MPC_Experiments_2/Simulate Plant Dynamics/x_dot -> x5/Hold this value ==
  In1 : Inport
  Action Port : ActionPort  ActionPortLabel=if(u1 ~= 0)
  Out1 : Outport  VectorParamsAs1DForOutWhenUnconnected=off
  wires:
  In1/1 -> Out1/1

== system MPC_Experiments_2/Simulate Plant Dynamics/x_dot -> x6/Hold this value ==
  In1 : Inport
  Action Port : ActionPort  ActionPortLabel=if(u1 ~= 0)
  Out1 : Outport  VectorParamsAs1DForOutWhenUnconnected=off
  wires:
  In1/1 -> Out1/1

== system MPC_Experiments_2/Simulate Plant Dynamics/x_dot -> x7/Hold this value ==
  In1 : Inport
  Action Port : ActionPort  ActionPortLabel=if(u1 ~= 0)
  Out1 : Outport  VectorParamsAs1DForOutWhenUnconnected=off
  wires:
  In1/1 -> Out1/1

== system MPC_Experiments_2/Simulate Plant Dynamics/x_dot -> x8/Hold this value ==
  In1 : Inport
  Action Port : ActionPort  ActionPortLabel=if(u1 ~= 0)
  Out1 : Outport  VectorParamsAs1DForOutWhenUnconnected=off
  wires:
  In1/1 -> Out1/1

== system MPC_Experiments_2/Simulate Plant Dynamics/x_dot -> x9/Hold this value ==
  In1 : Inport
  Action Port : ActionPort  ActionPortLabel=if(u1 ~= 0)
  Out1 : Outport  VectorParamsAs1DForOutWhenUnconnected=off
  wires:
  In1/1 -> Out1/1

== system MPC_Experiments_2/From Force//Torque to PWM Signal/Change BLACK Behavior/Calculate Thruster ON//OFF/Rotate Forces to Inertial ==
  "F_b " : Inport
  Rz : Inport  Port=2
  Create Rotation Matrix : MATLAB Function  TreatAsAtomicUnit=on
  Rotate F_b to F_I : Product  Multiplication=Matrix(*)
  F_I : Outport  VectorParamsAs1DForOutWhenUnconnected=off
  wires:
  "F_b "/1 -> Rotate F_b to F_I/2
  Rotate F_b to F_I/1 -> F_I/1
  Create Rotation Matrix/1(C_Ib) -> Rotate F_b to F_I/1
  Rz/1 -> Create Rotation Matrix/1(Rz)

== system MPC_Experiments_2/From Force//Torque to PWM Signal/Change BLACK Behavior/Calculate Thruster ON//OFF/pseudo-inverse ==
  H : Inport
  Product : Product  Multiplication=Matrix(*)
  Product1 : Product  Inputs=/  Multiplication=Matrix(*)
  Product2 : Product  Multiplication=Matrix(*)
  transpose : PermuteDimensions
  invH : Outport  VectorParamsAs1DForOutWhenUnconnected=off
  wires:
  Product2/1 -> invH/1
  transpose/1 -> Product/2, Product2/1
  Product/1 -> Product1/1
  H/1 -> Product/1, transpose/1
  Product1/1 -> Product2/2

== system MPC_Experiments_2/From Force//Torque to PWM Signal/Change BLUE Behavior/Calculate Thruster ON//OFF/Rotate Forces to Inertial ==
  "F_b " : Inport
  Rz : Inport  Port=2
  Create Rotation Matrix : MATLAB Function  TreatAsAtomicUnit=on
  Rotate F_b to F_I : Product  Multiplication=Matrix(*)
  F_I : Outport  VectorParamsAs1DForOutWhenUnconnected=off
  wires:
  "F_b "/1 -> Rotate F_b to F_I/2
  Rotate F_b to F_I/1 -> F_I/1
  Create Rotation Matrix/1(C_Ib) -> Rotate F_b to F_I/1
  Rz/1 -> Create Rotation Matrix/1(Rz)

== system MPC_Experiments_2/From Force//Torque to PWM Signal/Change BLUE Behavior/Calculate Thruster ON//OFF/pseudo-inverse ==
  H : Inport
  Product : Product  Multiplication=Matrix(*)
  Product1 : Product  Inputs=/  Multiplication=Matrix(*)
  Product2 : Product  Multiplication=Matrix(*)
  transpose : PermuteDimensions
  invH : Outport  VectorParamsAs1DForOutWhenUnconnected=off
  wires:
  Product2/1 -> invH/1
  transpose/1 -> Product/2, Product2/1
  Product/1 -> Product1/1
  H/1 -> Product/1, transpose/1
  Product1/1 -> Product2/2

== system MPC_Experiments_2/From Force//Torque to PWM Signal/Change RED Behavior/Calculate Thruster ON//OFF/Rotate Forces to Inertial ==
  "F_b " : Inport
  Rz : Inport  Port=2
  Create Rotation Matrix : MATLAB Function  TreatAsAtomicUnit=on
  Rotate F_b to F_I : Product  Multiplication=Matrix(*)
  F_I : Outport  VectorParamsAs1DForOutWhenUnconnected=off
  wires:
  "F_b "/1 -> Rotate F_b to F_I/2
  Rotate F_b to F_I/1 -> F_I/1
  Create Rotation Matrix/1(C_Ib) -> Rotate F_b to F_I/1
  Rz/1 -> Create Rotation Matrix/1(Rz)

== system MPC_Experiments_2/From Force//Torque to PWM Signal/Change RED Behavior/Calculate Thruster ON//OFF/pseudo-inverse ==
  H : Inport
  Product : Product  Multiplication=Matrix(*)
  Product1 : Product  Inputs=/  Multiplication=Matrix(*)
  Product2 : Product  Multiplication=Matrix(*)
  transpose : PermuteDimensions
  invH : Outport  VectorParamsAs1DForOutWhenUnconnected=off
  wires:
  Product2/1 -> invH/1
  transpose/1 -> Product/2, Product2/1
  Product/1 -> Product1/1
  H/1 -> Product/1, transpose/1
  Product1/1 -> Product2/2

== system MPC_Experiments_2/From Torque, Command RW/Change RED Behavior/Wheel RPM to PWM/Convert Wheel Rate to Motor Rate ==
  Wheel RPM : Inport
  Divide : Product  Inputs=**
  Gearbox Ratio : Constant  Value=3375/64
  Motor RPM : Outport  VectorParamsAs1DForOutWhenUnconnected=off
  wires:
  Gearbox Ratio/1 -> Divide/2
  Divide/1 -> Motor RPM/1
  Wheel RPM/1 -> Divide/1

== system MPC_Experiments_2/From Torque, Command RW/Change RED Behavior/Wheel RPM to PWM/Delay Bank ==
  Status : Inport
  Delay1 : Delay  DelayLength=1  InitialCondition=0
  Delay2 : Delay  InitialCondition=0
  Delay3 : Delay  DelayLength=4  InitialCondition=0
  Delay4 : Delay  DelayLength=5  InitialCondition=0
  Delay5 : Delay  DelayLength=3  InitialCondition=0
  Mostly zeros? : MinMax  Inputs=6
  StatusVector : Outport  VectorParamsAs1DForOutWhenUnconnected=off
  wires:
  Delay3/1 -> Mostly zeros?/5
  Status/1 -> Delay4/1, Delay3/1, Delay5/1, Delay2/1, Delay1/1, Mostly zeros?/1
  Delay2/1 -> Mostly zeros?/3
  Delay4/1 -> Mostly zeros?/6
  Delay5/1 -> Mostly zeros?/4
  Mostly zeros?/1 -> StatusVector/1
  Delay1/1 -> Mostly zeros?/2

== system MPC_Experiments_2/From Torque, Command RW/Change RED Behavior/Wheel RPM to PWM/Obtain RW Status ==
  GPIO Read1 : embdlinuxlib/GPIO Read  board=Pi 3 Model B  gpio=24  internalResistor=Off  sampleTime=0.1  direction=Input  blockPlatform=Raspberry Pi
      settings: SourceProductBaseCode=SC_BEAGLEBONE_BLUE,RASPPI
  RW_Status : Outport  VectorParamsAs1DForOutWhenUnconnected=off
  wires:
  GPIO Read1/1 -> RW_Status/1

== system MPC_Experiments_2/From Torque, Command RW/Change RED Behavior/Wheel RPM to PWM/Send Direction to Motor Controller ==
  WheelDir : Inport
  GPIO Write : embdlinuxlib/GPIO Write  board=Pi 3 Model B  gpio=21  direction=Output  blockPlatform=Raspberry Pi
      settings: SourceProductBaseCode=SC_BEAGLEBONE_BLUE,RASPPI
  wires:
  WheelDir/1 -> GPIO Write/1

== system MPC_Experiments_2/From Torque, Command RW/Change RED Behavior/Wheel RPM to PWM/Send PWM to Motor Controller ==
  MotorPWM : Inport
  PWM1 : raspberrypiBasiclib/PWM  board=Pi 3 Model B  Pin_=18  Frequency=10  blockPlatform=Raspberry Pi
      settings: SourceProductBaseCode=RASPPI
  wires:
  MotorPWM/1 -> PWM1/1

== system MPC_Experiments_2/From Torque, Command RW/Change RED Behavior/Wheel RPM to PWM/Turn on Motor ==
  EnableSig : Inport
  GPIO Write1 : embdlinuxlib/GPIO Write  board=Pi 3 Model B  gpio=25  direction=Output  blockPlatform=Raspberry Pi
      settings: SourceProductBaseCode=SC_BEAGLEBONE_BLUE,RASPPI
  wires:
  EnableSig/1 -> GPIO Write1/1

== system MPC_Experiments_2/Grab PhaseSpace Data via UDP/Use Hardware to Obtain States/Using RED+BLACK, or RED+BLACK+ARM/Is this a simulation? ==
  Constant : Constant  Value=simMode  SampleTime=-1
  isSim : Outport  VectorParamsAs1DForOutWhenUnconnected=off
  wires:
  Constant/1 -> isSim/1

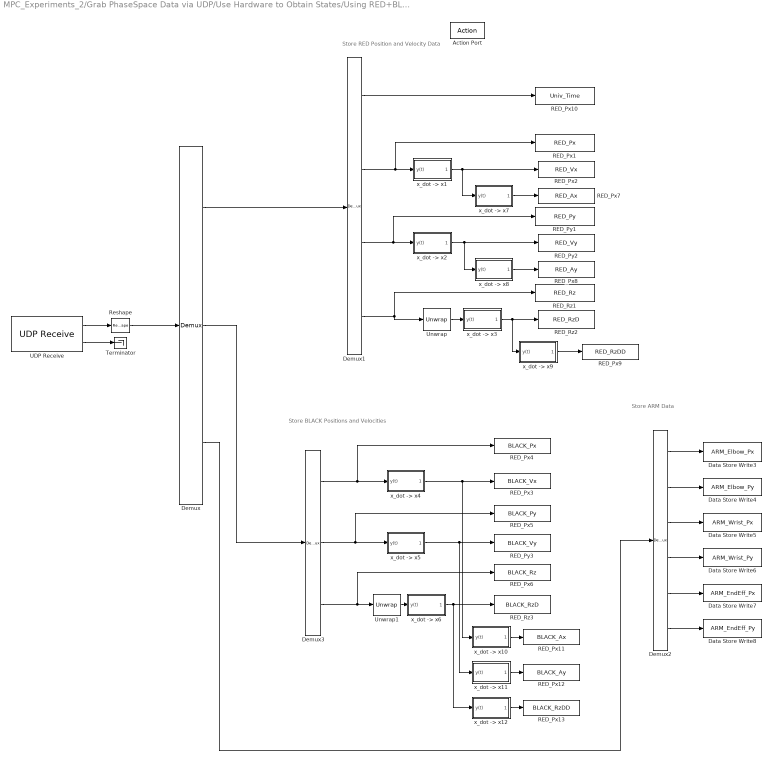
== system MPC_Experiments_2/Grab PhaseSpace Data via UDP/Use Hardware to Obtain States/Using RED+BLACK, or RED+BLACK+ARM/Obtain BLACK States ==
  note: Store ARM Data
  note: Store RED Position and Velocity Data
  note: Store BLACK Positions and Velocities
  Action Port : ActionPort  ActionPortLabel=if(u1 == 2 | u2 == 1)
  Data Store Write3 : DataStoreWrite  DataStoreName=ARM_Elbow_Px
  Data Store Write4 : DataStoreWrite  DataStoreName=ARM_Elbow_Py
  Data Store Write5 : DataStoreWrite  DataStoreName=ARM_Wrist_Px
  Data Store Write6 : DataStoreWrite  DataStoreName=ARM_Wrist_Py
  Data Store Write7 : DataStoreWrite  DataStoreName=ARM_EndEff_Px
  Data Store Write8 : DataStoreWrite  DataStoreName=ARM_EndEff_Py
  Demux : Demux  Outputs=[4,3,6]
  Demux1 : Demux
  Demux2 : Demux  Outputs=6
  Demux3 : Demux  Outputs=3
  RED_Px1 : DataStoreWrite  DataStoreName=RED_Px
  RED_Px10 : DataStoreWrite  DataStoreName=Univ_Time
  RED_Px11 : DataStoreWrite  DataStoreName=BLACK_Ax
  RED_Px12 : DataStoreWrite  DataStoreName=BLACK_Ay
  RED_Px13 : DataStoreWrite  DataStoreName=BLACK_RzDD
  RED_Px2 : DataStoreWrite  DataStoreName=RED_Vx
  RED_Px3 : DataStoreWrite  DataStoreName=BLACK_Vx
  RED_Px4 : DataStoreWrite  DataStoreName=BLACK_Px
  RED_Px5 : DataStoreWrite  DataStoreName=BLACK_Py
  RED_Px6 : DataStoreWrite  DataStoreName=BLACK_Rz
  RED_Px7 : DataStoreWrite  DataStoreName=RED_Ax
  RED_Px8 : DataStoreWrite  DataStoreName=RED_Ay
  RED_Px9 : DataStoreWrite  DataStoreName=RED_RzDD
  RED_Py1 : DataStoreWrite  DataStoreName=RED_Py
  RED_Py2 : DataStoreWrite  DataStoreName=RED_Vy
  RED_Py3 : DataStoreWrite  DataStoreName=BLACK_Vy
  RED_Rz1 : DataStoreWrite  DataStoreName=RED_Rz
  RED_Rz2 : DataStoreWrite  DataStoreName=RED_RzD
  RED_Rz3 : DataStoreWrite  DataStoreName=BLACK_RzD
  Reshape : Reshape  OutputDimensionality=Customize  OutputDimensions=[13,1]
  Terminator : Terminator
  UDP Receive : embdlinuxlib/UDP Receive  localURL='0.0.0.0'  localPort=25000  remoteURL='0.0.0.0'  remotePort=-1  recvBufferSize=8192  signalDatatype=double  dims=13  isVarSize=off  showBlockingTime=off  blockingTime=0  sampletime=-1  blockPlatform=Raspberry Pi
      settings: SourceProductBaseCode=SC_BEAGLEBONE_BLUE,RASPPI
  Unwrap : dspsigops/Unwrap  tol=pi  InputProcessing=Columns as channels (frame based)  running=off
  Unwrap1 : dspsigops/Unwrap  tol=pi  InputProcessing=Columns as channels (frame based)  running=off
  "x_dot -> x1" : Subsystem
  "x_dot -> x10" : Subsystem
  "x_dot -> x11" : Subsystem
  "x_dot -> x12" : Subsystem
  "x_dot -> x2" : Subsystem
  "x_dot -> x3" : Subsystem
  "x_dot -> x4" : Subsystem
  "x_dot -> x5" : Subsystem
  "x_dot -> x6" : Subsystem
  "x_dot -> x7" : Subsystem
  "x_dot -> x8" : Subsystem
  "x_dot -> x9" : Subsystem
  wires:
  UDP Receive/1 -> Reshape/1
  UDP Receive/2 -> Terminator/1
  "x_dot -> x8"/1(dy(t)/dt) -> RED_Px8/1
  Demux2/2 -> Data Store Write4/1
  Reshape/1 -> Demux/1
  Demux1/4 -> Unwrap/1, RED_Rz1/1
  Demux1/1 -> RED_Px10/1
  Unwrap/1 -> "x_dot -> x3"/1(y(t))
  "x_dot -> x7"/1(dy(t)/dt) -> RED_Px7/1
  Demux/2 -> Demux3/1
  "x_dot -> x9"/1(dy(t)/dt) -> RED_Px9/1
  Demux/1 -> Demux1/1
  Demux/3 -> Demux2/1
  "x_dot -> x3"/1(dy(t)/dt) -> "x_dot -> x9"/1(y(t)), RED_Rz2/1
  "x_dot -> x1"/1(dy(t)/dt) -> "x_dot -> x7"/1(y(t)), RED_Px2/1
  Demux1/2 -> "x_dot -> x1"/1(y(t)), RED_Px1/1
  Demux2/4 -> Data Store Write6/1
  Demux2/6 -> Data Store Write8/1
  "x_dot -> x2"/1(dy(t)/dt) -> "x_dot -> x8"/1(y(t)), RED_Py2/1
  Demux2/3 -> Data Store Write5/1
  Demux1/3 -> "x_dot -> x2"/1(y(t)), RED_Py1/1
  Demux2/1 -> Data Store Write3/1
  Demux2/5 -> Data Store Write7/1
  "x_dot -> x11"/1(dy(t)/dt) -> RED_Px12/1
  Demux3/2 -> "x_dot -> x5"/1(y(t)), RED_Px5/1
  Demux3/3 -> Unwrap1/1, RED_Px6/1
  "x_dot -> x5"/1(dy(t)/dt) -> RED_Py3/1, "x_dot -> x11"/1(y(t))
  "x_dot -> x4"/1(dy(t)/dt) -> "x_dot -> x10"/1(y(t)), RED_Px3/1
  "x_dot -> x6"/1(dy(t)/dt) -> RED_Rz3/1, "x_dot -> x12"/1(y(t))
  Unwrap1/1 -> "x_dot -> x6"/1(y(t))
  "x_dot -> x12"/1(dy(t)/dt) -> RED_Px13/1
  Demux3/1 -> "x_dot -> x4"/1(y(t)), RED_Px4/1
  "x_dot -> x10"/1(dy(t)/dt) -> RED_Px11/1

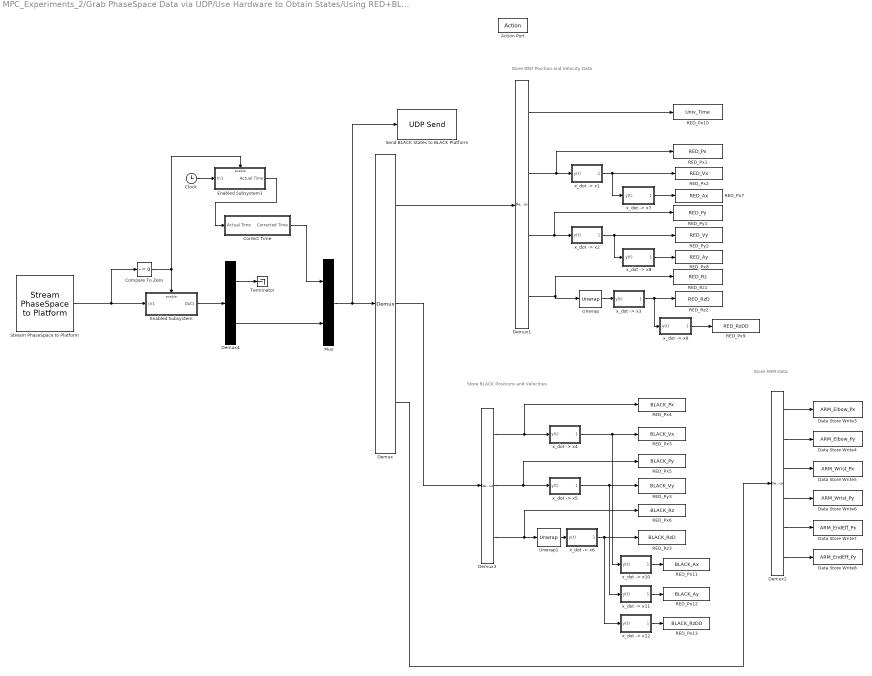
== system MPC_Experiments_2/Grab PhaseSpace Data via UDP/Use Hardware to Obtain States/Using RED+BLACK, or RED+BLACK+ARM/Obtain RED States ==
  note: Store ARM Data
  note: Store RED Position and Velocity Data
  note: Store BLACK Positions and Velocities
  Action Port : ActionPort  ActionPortLabel=if(u1 == 1 | u2 == 1)
  Clock : Clock
  Compare To Zero : simulink/Logic and Bit Operations/Compare To Zero  relop=~=  OutDataTypeStr=boolean
  Correct Time : Subsystem
  Data Store Write3 : DataStoreWrite  DataStoreName=ARM_Elbow_Px
  Data Store Write4 : DataStoreWrite  DataStoreName=ARM_Elbow_Py
  Data Store Write5 : DataStoreWrite  DataStoreName=ARM_Wrist_Px
  Data Store Write6 : DataStoreWrite  DataStoreName=ARM_Wrist_Py
  Data Store Write7 : DataStoreWrite  DataStoreName=ARM_EndEff_Px
  Data Store Write8 : DataStoreWrite  DataStoreName=ARM_EndEff_Py
  Demux : Demux  Outputs=[4,3,6]
  Demux1 : Demux
  Demux2 : Demux  Outputs=6
  Demux3 : Demux  Outputs=3
  Demux4 : Demux  Outputs=[1,12]
  Enabled Subsystem : Subsystem  TreatAsAtomicUnit=on
  Enabled Subsystem1 : Subsystem  TreatAsAtomicUnit=on
  Mux : Mux  Inputs=2
  RED_Px1 : DataStoreWrite  DataStoreName=RED_Px
  RED_Px10 : DataStoreWrite  DataStoreName=Univ_Time
  RED_Px11 : DataStoreWrite  DataStoreName=BLACK_Ax
  RED_Px12 : DataStoreWrite  DataStoreName=BLACK_Ay
  RED_Px13 : DataStoreWrite  DataStoreName=BLACK_RzDD
  RED_Px2 : DataStoreWrite  DataStoreName=RED_Vx
  RED_Px3 : DataStoreWrite  DataStoreName=BLACK_Vx
  RED_Px4 : DataStoreWrite  DataStoreName=BLACK_Px
  RED_Px5 : DataStoreWrite  DataStoreName=BLACK_Py
  RED_Px6 : DataStoreWrite  DataStoreName=BLACK_Rz
  RED_Px7 : DataStoreWrite  DataStoreName=RED_Ax
  RED_Px8 : DataStoreWrite  DataStoreName=RED_Ay
  RED_Px9 : DataStoreWrite  DataStoreName=RED_RzDD
  RED_Py1 : DataStoreWrite  DataStoreName=RED_Py
  RED_Py2 : DataStoreWrite  DataStoreName=RED_Vy
  RED_Py3 : DataStoreWrite  DataStoreName=BLACK_Vy
  RED_Rz1 : DataStoreWrite  DataStoreName=RED_Rz
  RED_Rz2 : DataStoreWrite  DataStoreName=RED_RzD
  RED_Rz3 : DataStoreWrite  DataStoreName=BLACK_RzD
  Send BLACK States to BLACK Platform : embdlinuxlib/UDP Send  remoteURL='192.168.0.101'  remotePort=25000  localURL='255.255.255.255'  localPortSource=Automatically determine  localPort=-1  sampletime=-1  blockPlatform=Raspberry Pi  separateLengthPort=0
      settings: SourceProductBaseCode=SC_BEAGLEBONE_BLUE,RASPPI
  Stream PhaseSpace to Platform : MainLibrary/PhaseSpace Functions/Stream PhaseSpace to Platform  platformSelection=platformSelection  PS_SampleRate=1/serverRate
      settings: SourceProductName=SPOT Custom Library
  Terminator : Terminator
  Unwrap : dspsigops/Unwrap  tol=pi  InputProcessing=Columns as channels (frame based)  running=off
  Unwrap1 : dspsigops/Unwrap  tol=pi  InputProcessing=Columns as channels (frame based)  running=off
  "x_dot -> x1" : Subsystem
  "x_dot -> x10" : Subsystem
  "x_dot -> x11" : Subsystem
  "x_dot -> x12" : Subsystem
  "x_dot -> x2" : Subsystem
  "x_dot -> x3" : Subsystem
  "x_dot -> x4" : Subsystem
  "x_dot -> x5" : Subsystem
  "x_dot -> x6" : Subsystem
  "x_dot -> x7" : Subsystem
  "x_dot -> x8" : Subsystem
  "x_dot -> x9" : Subsystem
  wires:
  "x_dot -> x8"/1(dy(t)/dt) -> RED_Px8/1
  Demux2/2 -> Data Store Write4/1
  Demux1/4 -> Unwrap/1, RED_Rz1/1
  Demux1/1 -> RED_Px10/1
  Unwrap/1 -> "x_dot -> x3"/1(y(t))
  "x_dot -> x7"/1(dy(t)/dt) -> RED_Px7/1
  Demux/2 -> Demux3/1
  "x_dot -> x9"/1(dy(t)/dt) -> RED_Px9/1
  Demux/1 -> Demux1/1
  Demux/3 -> Demux2/1
  "x_dot -> x3"/1(dy(t)/dt) -> "x_dot -> x9"/1(y(t)), RED_Rz2/1
  "x_dot -> x1"/1(dy(t)/dt) -> "x_dot -> x7"/1(y(t)), RED_Px2/1
  Demux1/2 -> "x_dot -> x1"/1(y(t)), RED_Px1/1
  Demux2/4 -> Data Store Write6/1
  Demux2/6 -> Data Store Write8/1
  "x_dot -> x2"/1(dy(t)/dt) -> "x_dot -> x8"/1(y(t)), RED_Py2/1
  Demux2/3 -> Data Store Write5/1
  Demux1/3 -> "x_dot -> x2"/1(y(t)), RED_Py1/1
  Demux2/1 -> Data Store Write3/1
  Demux2/5 -> Data Store Write7/1
  "x_dot -> x11"/1(dy(t)/dt) -> RED_Px12/1
  Demux3/2 -> "x_dot -> x5"/1(y(t)), RED_Px5/1
  Demux3/3 -> Unwrap1/1, RED_Px6/1
  "x_dot -> x5"/1(dy(t)/dt) -> RED_Py3/1, "x_dot -> x11"/1(y(t))
  "x_dot -> x4"/1(dy(t)/dt) -> "x_dot -> x10"/1(y(t)), RED_Px3/1
  "x_dot -> x6"/1(dy(t)/dt) -> RED_Rz3/1, "x_dot -> x12"/1(y(t))
  Unwrap1/1 -> "x_dot -> x6"/1(y(t))
  "x_dot -> x12"/1(dy(t)/dt) -> RED_Px13/1
  Demux3/1 -> "x_dot -> x4"/1(y(t)), RED_Px4/1
  "x_dot -> x10"/1(dy(t)/dt) -> RED_Px11/1
  Enabled Subsystem1/1(Actual Time) -> Correct Time/1(Actual Time)
  Demux4/1 -> Terminator/1
  Correct Time/1(Corrected Time) -> Mux/1
  Clock/1 -> Enabled Subsystem1/1(In1)
  Stream PhaseSpace to Platform/1 -> Enabled Subsystem/1(In1), Compare To Zero/1
  Compare To Zero/1 -> Enabled Subsystem1/Enable, Enabled Subsystem/Enable
  Demux4/2 -> Mux/2
  Enabled Subsystem/1(Out1) -> Demux4/1
  Mux/1 -> Send BLACK States to BLACK Platform/1, Demux/1

== system MPC_Experiments_2/Grab PhaseSpace Data via UDP/Use Hardware to Obtain States/Using RED, BLACK, BLUE, or RED + ARM/Correct Time ==
  Actual Time : Inport
  Edge Detector : dspswit3/Edge Detector  InputProcessing=Columns as channels (frame based)
      settings: SourceProductBaseCode=DS
  Enabled Subsystem : Subsystem  TreatAsAtomicUnit=on
  Subtract : Sum  Inputs=+-
  Corrected Time : Outport  VectorParamsAs1DForOutWhenUnconnected=off
  wires:
  Subtract/1 -> Corrected Time/1
  Edge Detector/1 -> Enabled Subsystem/Enable
  Actual Time/1 -> Subtract/1, Enabled Subsystem/1(In1), Edge Detector/1
  Enabled Subsystem/1(Out1) -> Subtract/2

== system MPC_Experiments_2/Grab PhaseSpace Data via UDP/Use Hardware to Obtain States/Using RED, BLACK, BLUE, or RED + ARM/Enabled Subsystem ==
  In1 : Inport
  Enable : EnablePort
  Out1 : Outport  VectorParamsAs1DForOutWhenUnconnected=off
  wires:
  In1/1 -> Out1/1

== system MPC_Experiments_2/Grab PhaseSpace Data via UDP/Use Hardware to Obtain States/Using RED, BLACK, BLUE, or RED + ARM/Enabled Subsystem1 ==
  In1 : Inport
  Enable : EnablePort
  Actual Time : Outport  VectorParamsAs1DForOutWhenUnconnected=off
  wires:
  In1/1 -> Actual Time/1

== system MPC_Experiments_2/Grab PhaseSpace Data via UDP/Use Hardware to Obtain States/Using RED, BLACK, BLUE, or RED + ARM/x_dot -> x1 ==
  note: dy/dt ~= (y2-y1)/deltaT
  y(t) : Inport
  Delay1 : Delay  DelayLength=1  InitialConditionSource=Input port
      settings: InputPortMap=u0,p4
  Hold this value : Subsystem  TreatAsAtomicUnit=on
  Sum6 : Sum  Inputs=-+|
  divide by delta T : Gain  Gain=1/serverRate
  "if we went through a \"step\"" : If  IfExpression=u1 ~= 0  ShowElse=off
  dy(t)/dt : Outport  VectorParamsAs1DForOutWhenUnconnected=off
  wires:
  divide by delta T/1 -> dy(t)/dt/1
  Delay1/1 -> Sum6/1
  "if we went through a \"step\""/1 -> Hold this value/Action
  Hold this value/1(Out1) -> divide by delta T/1
  Sum6/1 -> "if we went through a \"step\""/1, Hold this value/1(In1)
  y(t)/1 -> Sum6/2, Delay1/2, Delay1/1
